simulink model "zad1v1"  (R2014b)
settings: Solver=ode45  StartTime=0.0  StopTime=70  RelTol=1e-3
values from neighbouring files (symbols this model uses):
  a1 = -0.28    [set_params.m]
  a2 = -0.9    [set_params.m]
  a3 = 0.35    [set_params.m]
  a4 = 0.3    [set_params.m]
  K = 4.5    [set_params.m]
  T1 = 5    [set_params.m]
  T2 = 8    [set_params.m]
settings Model: Creator=kuba  LastModifiedBy=kuba
settings DebuggingCC: SolverPrmCheckMsg=none

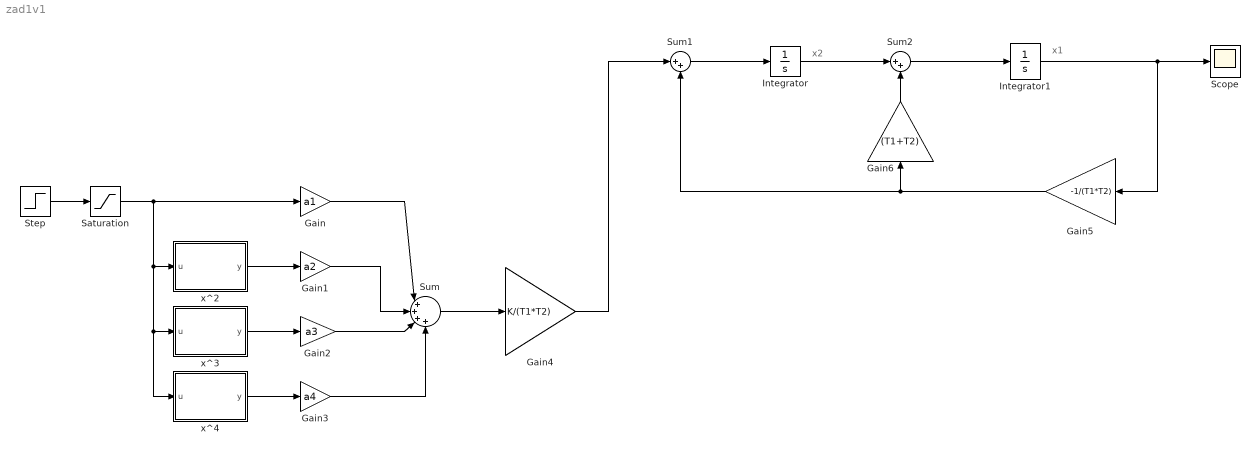
== system zad1v1 ==
  note: x2
  note: x1
  Gain : Gain  Gain=a1
  Gain1 : Gain  Gain=a2
  Gain2 : Gain  Gain=a3
  Gain3 : Gain  Gain=a4
  Gain4 : Gain  Gain=K/(T1*T2)
  Gain5 : Gain  Gain=-1/(T1*T2)
  Gain6 : Gain  Gain=(T1+T2)
  Integrator : Integrator
  Integrator1 : Integrator
  Saturation : Saturate  UpperLimit=1  LowerLimit=-1
  Scope : Scope
  Step : Step  SampleTime=0
  Sum : Sum  Inputs=|++++
  Sum1 : Sum  Inputs=|++
  Sum2 : Sum  Inputs=|++
  x^2 : MATLAB Function  TreatAsAtomicUnit=on
  x^3 : MATLAB Function  TreatAsAtomicUnit=on
  x^4 : MATLAB Function  TreatAsAtomicUnit=on
  wires:
  Saturation/1 -> x^4/1(u), x^3/1(u), x^2/1(u), Gain/1
  x^2/1(y) -> Gain1/1
  x^3/1(y) -> Gain2/1
  x^4/1(y) -> Gain3/1
  Gain/1 -> Sum/1
  Gain1/1 -> Sum/2
  Gain2/1 -> Sum/3
  Gain3/1 -> Sum/4
  Sum/1 -> Gain4/1
  Gain4/1 -> Sum1/1
  Sum2/1 -> Integrator1/1
  Sum1/1 -> Integrator/1
  Integrator1/1 -> Gain5/1, Scope/1
  Gain5/1 -> Gain6/1, Sum1/2
  Gain6/1 -> Sum2/2
  Step/1 -> Saturation/1
  Integrator/1 -> Sum2/1

== matlab function zad1v1/x^3 ==
  data: u input; y output
function y = cube(u)
y = u^3;

== matlab function zad1v1/x^2 ==
  data: u input; y output
function y = square(u)
y = u^2;

== matlab function zad1v1/x^4 ==
  data: u input; y output
function y = quad(u)
y = u^4;
